simulink model "Telerobotic_System_With_Delay"  (R2020a)
settings: Solver=VariableStepAuto  StartTime=0.0  StopTime=10.0  RelTol=1e-3
values from neighbouring files (symbols this model uses):
  B = 1 / k_m    (= 0.0517063081696)    [Teleop_parameters.m]    (also in base.mat; base_no_attrito.mat = 0; ci_siamo.mat; force_control.mat)
  Be = 5    [Teleop_parameters.m]    (also in base.mat = 0.5; base_no_attrito.mat = 0.5; ci_siamo.mat; force_control.mat = 0.5)
  Bh = 0.02    [Teleop_parameters.m]    (also in base.mat; base_no_attrito.mat; ci_siamo.mat; force_control.mat)
  Fc_h = 5    [Teleop_parameters.m]    (also in base.mat; base_no_attrito.mat; ci_siamo.mat; force_control.mat)
  J = tau_m / k_m    (= 0.0629265770424)    [Teleop_parameters.m]    (also in base.mat; base_no_attrito.mat; ci_siamo.mat; force_control.mat)
  Jh = 0.02    [Teleop_parameters.m]    (also in base.mat; base_no_attrito.mat; ci_siamo.mat; force_control.mat)
  Kc2v_m = 2    [Teleop_parameters.m]    (also in base.mat; base_no_attrito.mat; ci_siamo.mat; force_control.mat)
  Kc2v_s = 2    [Teleop_parameters.m]    (also in base.mat; base_no_attrito.mat; ci_siamo.mat; force_control.mat)
  Kd_h = 1    [Teleop_parameters.m]    (also in base.mat; base_no_attrito.mat; ci_siamo.mat = 10; force_control.mat)
  Kd_s = 1    [Teleop_parameters.m]    (also in base.mat; base_no_attrito.mat; ci_siamo.mat = 0.5; force_control.mat)
  Ke = 10    [Teleop_parameters.m]    (also in base.mat; base_no_attrito.mat; ci_siamo.mat; force_control.mat)
  Kp_h = 1.2    [Teleop_parameters.m]    (also in base.mat; base_no_attrito.mat; ci_siamo.mat = 10; force_control.mat)
  Kp_s = 1    [Teleop_parameters.m]    (also in base.mat; base_no_attrito.mat; ci_siamo.mat; force_control.mat)
  Kt2c_m = 1.182    [Teleop_parameters.m]    (also in base.mat; base_no_attrito.mat; ci_siamo.mat; force_control.mat)
  Kt2c_s = 1.182    [Teleop_parameters.m]    (also in base.mat; base_no_attrito.mat; ci_siamo.mat; force_control.mat)
  lArm_m = 0.1    [Teleop_parameters.m]    (also in base.mat; base_no_attrito.mat; ci_siamo.mat; force_control.mat)
  lArm_s = 0.1    [Teleop_parameters.m]    (also in base.mat; base_no_attrito.mat; ci_siamo.mat; force_control.mat)
  maxCurrent_m = 4.5    [Teleop_parameters.m]    (also in base.mat; base_no_attrito.mat; ci_siamo.mat; force_control.mat)
  maxCurrent_s = 4.5    [Teleop_parameters.m]    (also in base.mat; base_no_attrito.mat; ci_siamo.mat; force_control.mat)
  qe = 5    [Teleop_parameters.m]    (also in base.mat; base_no_attrito.mat; ci_siamo.mat = 0.5; force_control.mat)
undefined symbols (not defined in the file or in its folder): Bl, Jl, Km, L, N, R
settings Model: Creator=giovanni  LastModifiedBy=giovanni

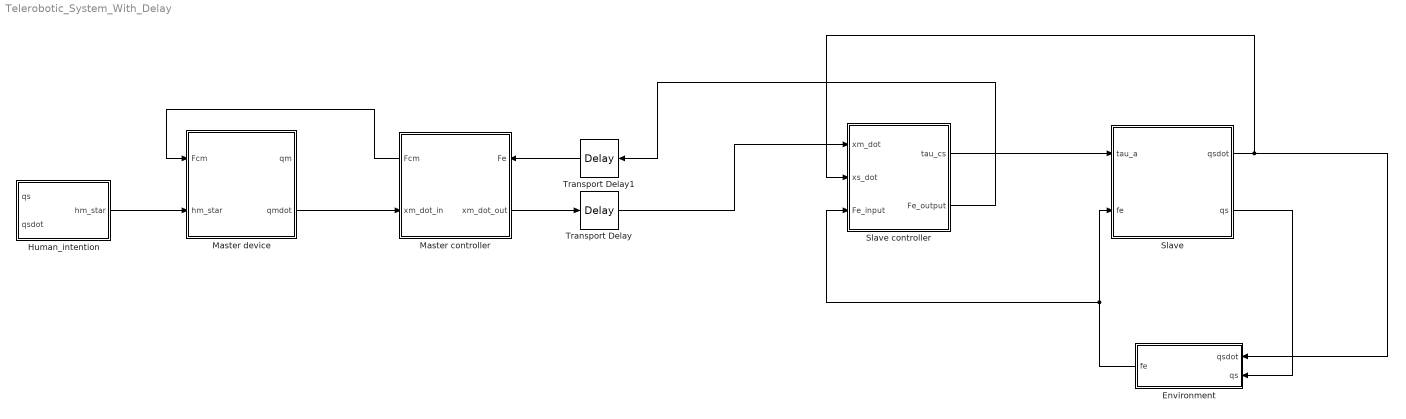
== system Telerobotic_System_With_Delay ==
  Environment : Subsystem
  Human_intention : Subsystem
  Master controller : Subsystem
      settings: PortSchema="{\"entries\":[{\"content\":{\"sides\":[{\"content\":{\"connectorIds\":[\"Out2\",\"In1\"]},\"type\":\"ConnectorPlacement.EquallySpacedRectSide\",\"uuid\":\"58cad0be-5678-476e-b9f4-5e642f2ef19b\"},{\"content\":{\"connectorIds\":[\"In2\",\"Out1\"],\"side\":\"RIGHT\"},\"type\":\"ConnectorPlacement.EquallySpacedRectSide\",\"uuid\":\"cc63c309-fcbf-4410-a336-38b734e557a5\"},{\"content\":{\"connectorIds\":[],\"side\":\"TOP\"},\"type\":\"ConnectorPlacement.EquallySpacedRectSide\",\"uuid\":\"ea1adacf-cd59-4cd0-a9d5-037ae620c70b\"}]},\"type\":\"ConnectorPlacement.EquallySpacedConnector\",\"uuid\":\"d7a720f5-56ec-42ad-98a9-cb46181e4957\"}],\"packageUris\":[\"http://schema.mathworks.com/mf0/Connector/19700101\"],\"version\":\"1.0\"}"
  Master device : Subsystem
  Slave : Subsystem
  Slave controller : Subsystem
  Transport Delay : TransportDelay
  Transport Delay1 : TransportDelay
  wires:
  Human_intention/1(hm_star) -> Master device/2(hm_star)
  Master controller/2(Fcm) -> Master device/1(Fcm)
  Master device/2(qmdot) -> Master controller/1(xm_dot_in)
  Master controller/1(xm_dot_out) -> Transport Delay/1
  Transport Delay1/1 -> Master controller/2(Fe)
  Slave controller/2(Fe_output) -> Transport Delay1/1
  Transport Delay/1 -> Slave controller/1(xm_dot)
  Slave controller/1(tau_cs) -> Slave/1(tau_a)
  Slave/1(qsdot) -> Environment/1(qsdot), Slave controller/2(xs_dot)
  Slave/2(qs) -> Environment/2(qs)
  Environment/1(fe) -> Slave controller/3(Fe_input), Slave/2(fe)

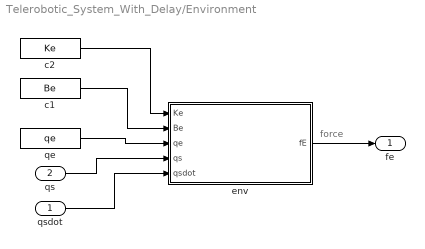
== system Telerobotic_System_With_Delay/Environment ==
  note: force
  qsdot : Inport
  qs : Inport  Port=2
  c1 : Constant  Value=Be  SampleTime=0
  c2 : Constant  Value=Ke  SampleTime=0
  env : MATLAB Function  TreatAsAtomicUnit=on
  qe : Constant  Value=qe  SampleTime=0
  fe : Outport  VectorParamsAs1DForOutWhenUnconnected=off
  wires:
  qe/1 -> env/3(qe)
  c1/1 -> env/2(Be)
  c2/1 -> env/1(Ke)
  qs/1 -> env/4(qs)
  qsdot/1 -> env/5(qsdot)
  env/1(fE) -> fe/1

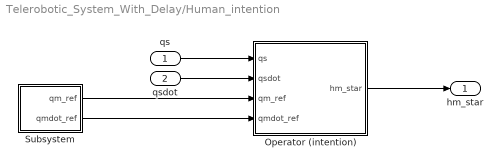
== system Telerobotic_System_With_Delay/Human_intention ==
  qs : Inport
  qsdot : Inport  Port=2
  Operator (intention) : Subsystem
  Subsystem : Subsystem
  hm_star : Outport
  wires:
  Subsystem/1(qm_ref) -> Operator (intention)/3(qm_ref)
  Subsystem/2(qmdot_ref) -> Operator (intention)/4(qmdot_ref)
  Operator (intention)/1(hm_star) -> hm_star/1
  qs/1 -> Operator (intention)/1(qs)
  qsdot/1 -> Operator (intention)/2(qsdot)

== system Telerobotic_System_With_Delay/Master controller ==
  xm_dot_in : Inport
  Fe : Inport  Port=2
  xm_dot_out : Outport
  Fcm : Outport  Port=2
  wires:
  Fe/1 -> Fcm/1
  xm_dot_in/1 -> xm_dot_out/1

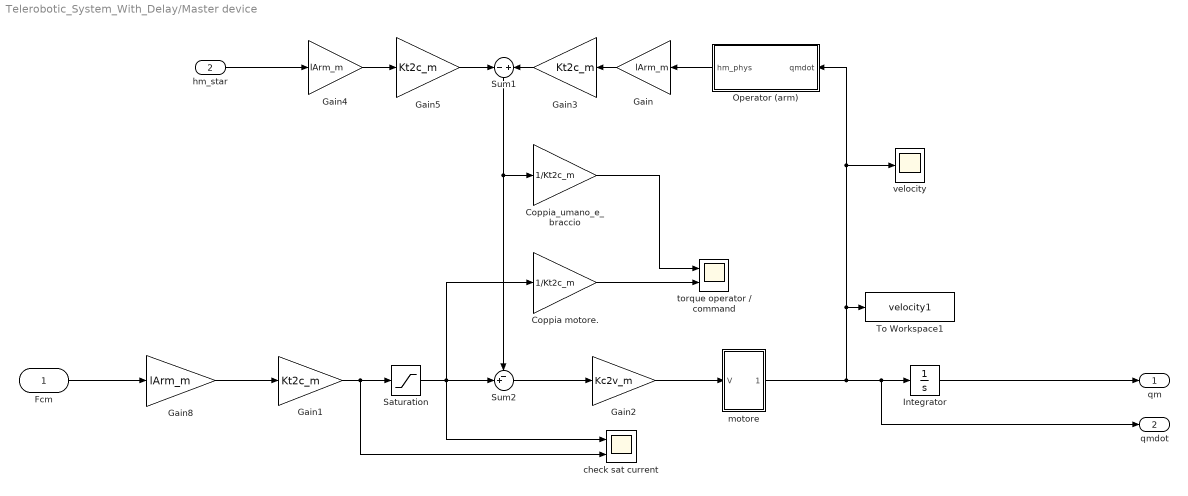
== system Telerobotic_System_With_Delay/Master device ==
  Fcm : Inport
  hm_star : Inport  Port=2
  Coppia motore. : Gain  Gain=1/Kt2c_m
  Coppia_umano_e_braccio : Gain  Gain=1/Kt2c_m
  Gain : Gain  Gain=lArm_m
  Gain1 : Gain  Gain=Kt2c_m
  Gain2 : Gain  Gain=Kc2v_m
  Gain3 : Gain  Gain=Kt2c_m
  Gain4 : Gain  Gain=lArm_m
  Gain5 : Gain  Gain=Kt2c_m
  Gain8 : Gain  Gain=lArm_m
  Integrator : Integrator
  Operator (arm) : Subsystem
  Saturation : Saturate  UpperLimit=maxCurrent_m  LowerLimit=-maxCurrent_m
  Sum1 : Sum  Inputs=-+
  Sum2 : Sum  Inputs=-+|
  To Workspace1 : ToWorkspace  VariableName=velocity1  SaveFormat=Timeseries  SampleTime=-1
  check sat current : Scope  NumInputPorts=2
  motore : Subsystem
  torque operator / command : Scope  NumInputPorts=2
  velocity : Scope
  qm : Outport
  qmdot : Outport  Port=2
  wires:
  Integrator/1 -> qm/1
  Sum2/1 -> Gain2/1
  Gain3/1 -> Sum1/2
  Gain2/1 -> motore/1(V)
  Gain1/1 -> check sat current/2, Saturation/1
  Coppia_umano_e_braccio/1 -> torque operator / command/1
  Coppia motore./1 -> torque operator / command/2
  motore/1(qdot) -> velocity/1, Operator (arm)/1(qmdot), To Workspace1/1, qmdot/1, Integrator/1
  Gain8/1 -> Gain1/1
  Gain5/1 -> Sum1/1
  Operator (arm)/1(hm_phys) -> Gain/1
  Sum1/1 -> Sum2/1, Coppia_umano_e_braccio/1
  Saturation/1 -> Coppia motore./1, Sum2/2, check sat current/1
  Gain/1 -> Gain3/1
  Gain4/1 -> Gain5/1
  Fcm/1 -> Gain8/1
  hm_star/1 -> Gain4/1

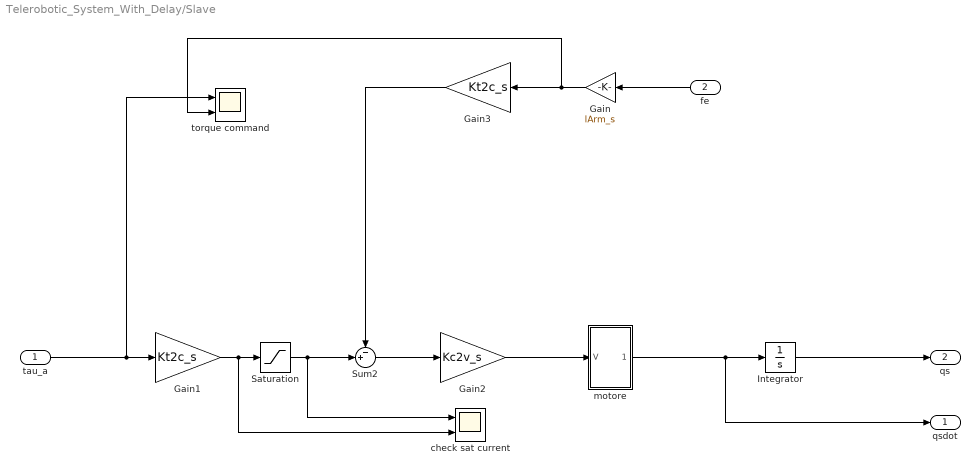
== system Telerobotic_System_With_Delay/Slave ==
  tau_a : Inport
  fe : Inport  Port=2
  Gain : Gain  Gain=lArm_s
  Gain1 : Gain  Gain=Kt2c_s
  Gain2 : Gain  Gain=Kc2v_s
  Gain3 : Gain  Gain=Kt2c_s
  Integrator : Integrator
  Saturation : Saturate  UpperLimit=maxCurrent_s  LowerLimit=-maxCurrent_s
  Sum2 : Sum  Inputs=-+|
  check sat current : Scope  NumInputPorts=2
  motore : Subsystem
  torque command : Scope  NumInputPorts=2
  qsdot : Outport
  qs : Outport  Port=2
  wires:
  Integrator/1 -> qs/1
  Sum2/1 -> Gain2/1
  Saturation/1 -> Sum2/2, check sat current/1
  Gain2/1 -> motore/1(V)
  Gain1/1 -> check sat current/2, Saturation/1
  Gain3/1 -> Sum2/1
  tau_a/1 -> torque command/1, Gain1/1
  fe/1 -> Gain/1
  Gain/1 -> torque command/2, Gain3/1
  motore/1(qdot) -> qsdot/1, Integrator/1

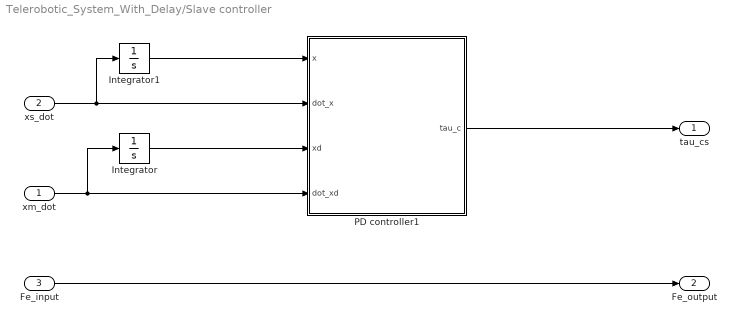
== system Telerobotic_System_With_Delay/Slave controller ==
  xm_dot : Inport
  xs_dot : Inport  Port=2
  Fe_input : Inport  Port=3
  Integrator : Integrator
  Integrator1 : Integrator
  PD controller1 : Subsystem
  tau_cs : Outport
  Fe_output : Outport  Port=2
  wires:
  Integrator/1 -> PD controller1/3(xd)
  xm_dot/1 -> PD controller1/4(dot_xd), Integrator/1
  PD controller1/1(tau_c) -> tau_cs/1
  Integrator1/1 -> PD controller1/1(x)
  xs_dot/1 -> Integrator1/1, PD controller1/2(dot_x)
  Fe_input/1 -> Fe_output/1

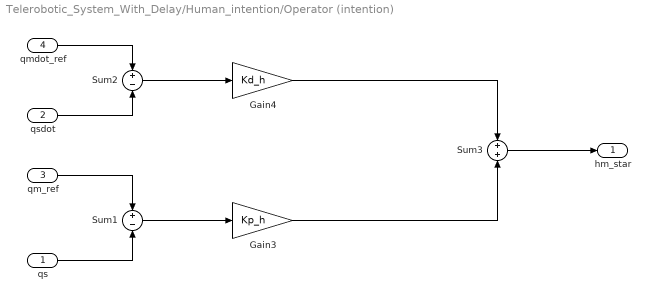
== system Telerobotic_System_With_Delay/Human_intention/Operator (intention) ==
  qs : Inport
  qsdot : Inport  Port=2
  qm_ref : Inport  Port=3
  qmdot_ref : Inport  Port=4
  Gain3 : Gain  Gain=Kp_h
  Gain4 : Gain  Gain=Kd_h
  Sum1 : Sum  Inputs=+|-
  Sum2 : Sum  Inputs=+|-
  Sum3 : Sum  Inputs=+|+
  hm_star : Outport  VectorParamsAs1DForOutWhenUnconnected=off
  wires:
  qs/1 -> Sum1/2
  qm_ref/1 -> Sum1/1
  qmdot_ref/1 -> Sum2/1
  Sum1/1 -> Gain3/1
  qsdot/1 -> Sum2/2
  Sum2/1 -> Gain4/1
  Gain4/1 -> Sum3/1
  Gain3/1 -> Sum3/2
  Sum3/1 -> hm_star/1

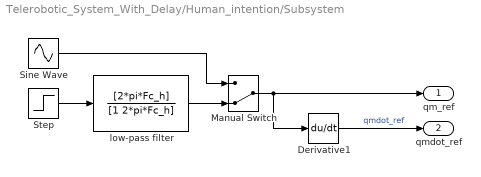
== system Telerobotic_System_With_Delay/Human_intention/Subsystem ==
  Derivative1 : Derivative  CoefficientInTFapproximation=0.001
  Manual Switch : ManualSwitch  CurrentSetting=0
  Sine Wave : Sin  SampleTime=0
  Step : Step  SampleTime=0
  low-pass filter : TransferFcn  Numerator=[2*pi*Fc_h]  Denominator=[1 2*pi*Fc_h]
  qm_ref : Outport
  qmdot_ref : Outport  Port=2
  wires:
  low-pass filter/1 -> Manual Switch/2
  Manual Switch/1 -> qm_ref/1, Derivative1/1
  Derivative1/1 -> qmdot_ref/1  "qmdot_ref"
  Step/1 -> low-pass filter/1
  Sine Wave/1 -> Manual Switch/1

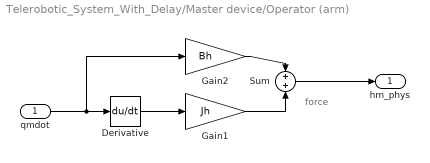
== system Telerobotic_System_With_Delay/Master device/Operator (arm) ==
  note: force
  qmdot : Inport
  Derivative : Derivative  CoefficientInTFapproximation=0.001
  Gain1 : Gain  Gain=Jh
  Gain2 : Gain  Gain=Bh
  Sum : Sum  Inputs=+|+
  hm_phys : Outport  VectorParamsAs1DForOutWhenUnconnected=off
  wires:
  qmdot/1 -> Gain2/1, Derivative/1
  Sum/1 -> hm_phys/1
  Derivative/1 -> Gain1/1
  Gain2/1 -> Sum/1
  Gain1/1 -> Sum/2

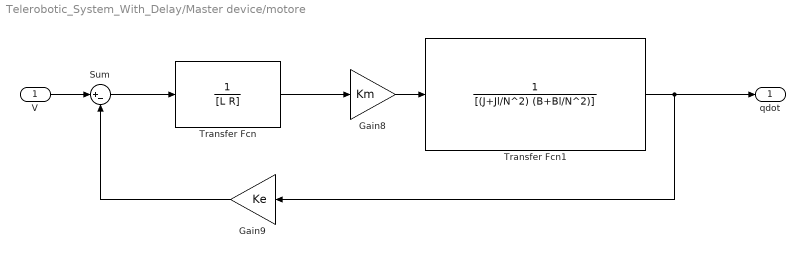
== system Telerobotic_System_With_Delay/Master device/motore ==
  V : Inport
  Gain8 : Gain  Gain=Km
  Gain9 : Gain  Gain=Ke
  Sum : Sum  Inputs=|+-
  Transfer Fcn : TransferFcn  Denominator=[L R]
  Transfer Fcn1 : TransferFcn  Denominator=[(J+Jl/N^2) (B+Bl/N^2)]
  qdot : Outport
  wires:
  Sum/1 -> Transfer Fcn/1
  V/1 -> Sum/1
  Transfer Fcn/1 -> Gain8/1
  Gain9/1 -> Sum/2
  Gain8/1 -> Transfer Fcn1/1
  Transfer Fcn1/1 -> Gain9/1, qdot/1

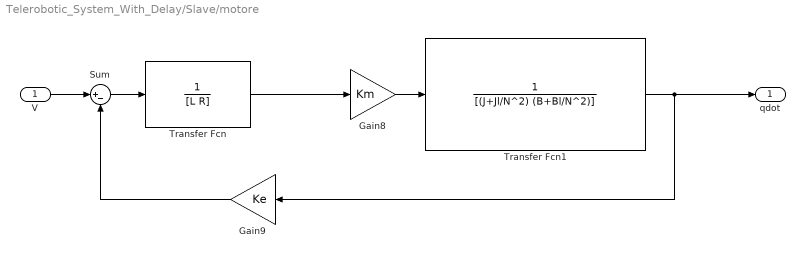
== system Telerobotic_System_With_Delay/Slave/motore ==
  V : Inport
  Gain8 : Gain  Gain=Km
  Gain9 : Gain  Gain=Ke
  Sum : Sum  Inputs=|+-
  Transfer Fcn : TransferFcn  Denominator=[L R]
  Transfer Fcn1 : TransferFcn  Denominator=[(J+Jl/N^2) (B+Bl/N^2)]
  qdot : Outport
  wires:
  Sum/1 -> Transfer Fcn/1
  V/1 -> Sum/1
  Transfer Fcn/1 -> Gain8/1
  Gain9/1 -> Sum/2
  Gain8/1 -> Transfer Fcn1/1
  Transfer Fcn1/1 -> Gain9/1, qdot/1

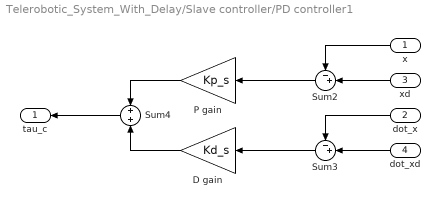
== system Telerobotic_System_With_Delay/Slave controller/PD controller1 ==
  x : Inport
  dot_x : Inport  Port=2
  xd : Inport  Port=3
  dot_xd : Inport  Port=4
  D gain : Gain  Gain=Kd_s
  P gain : Gain  Gain=Kp_s
  Sum2 : Sum  Inputs=-+|
  Sum3 : Sum  Inputs=-+|
  Sum4 : Sum
  tau_c : Outport  VectorParamsAs1DForOutWhenUnconnected=off
  wires:
  D gain/1 -> Sum4/2
  dot_x/1 -> Sum3/1
  dot_xd/1 -> Sum3/2
  x/1 -> Sum2/1
  xd/1 -> Sum2/2
  Sum3/1 -> D gain/1
  P gain/1 -> Sum4/1
  Sum4/1 -> tau_c/1
  Sum2/1 -> P gain/1

== matlab function Telerobotic_System_With_Delay/Environment/env ==
  data: Ke input; Be input; qe input; qs input; fE output; qsdot input
function fE  = environment(Ke, Be, qe, qs, qsdot)
if qs > qe
   fE = Ke * (qs - qe) + Be * qsdot;
else
   fE = 0;
end
